simulink model "pathFollowingSystemROS"  (R2020b)
settings: Solver=VariableStepAuto  StartTime=0.0  StopTime=inf  FixedStep=0.01  RelTol=1e-3  EnableMultiTasking=on
PreLoadFcn:
  | load('turtleBotMazeMap.mat')
  | [mapMatrix,mapResolution, mapOrigin] = convertMapToMatrix(myOccMap);
undefined symbols (not defined in the file or in its folder): Angular, Linear, mapMatrix, mapOrigin, mapResolution
libraries: robotlib x4, robotalgslib x2, robotcorelib x1
settings Model: EnablePacing=on  Creator=scastro  LastModifiedBy=josea
settings DataIOCC: LimitDataPoints=on  ReturnWorkspaceOutputs=off
settings OptimizationCC: LifeSpan=inf
settings DebuggingCC: AllowSymbolicDim=off  SFUnexpectedBacktrackingDiag=warning  SFNoUnconditionalDefaultTransitionDiag=warning  SFExecutionAtInitializationDiag=none  ArithmeticOperatorsInVariantConditions=warning
settings SFSimCC: SimUseLocalCustomCode=off  CustomCodeUndefinedFunction=UseInterfaceOnly
settings RTWCC: RTWUseLocalCustomCode=off
settings CodeAppCC: StateflowObjectComments=on
settings GRTTargetCC: TargetLangStandard=C89/C90 (ANSI)
settings ConfigComp: CovMetricSettings=dw  CovSaveCumulativeToWorkspaceVar=on  CovSaveSingleToWorkspaceVar=on  CovExternalEMLEnable=off  CovSFcnEnable=off
settings SimscapeCC: SimscapeNominalValues="[{\"value\":\"10\",\"unit\":\"V\"},{\"value\":\"1\",\"unit\":\"A\"},{\"value\":\"10\",\"unit\":\"N*m\"},{\"value\":\"10\",\"unit\":\"bar\"},{\"value\":\"100\",\"unit\":\"kJ/kg\"},{\"value\":\"1\",\"unit\":\"kW\"},{\"value\":\"300\",\"unit\":\"K\"},{\"value\":\"100\",\"unit\":\"cm^3/s\"},{\"value\":\"1\",\"unit\":\"kN\"},{\"value\":\"1\",\"unit\":\"g/cm^3\"},{\"value\":\"1\",\"unit\":\"l\"},{\"value\":\"1\",\"unit\":\"cm^2\"},{\"value\":\"60\",\"unit\":\"Hz\"}]"  SimscapeLogType=all  SimscapeLogDataHistory=10000
settings ConfigurationSet: Description=SimMechanics 2G
settings ExplorerConfigSet: InternalSimMechanicsExplorerSettings="<ExplorerConfiguration><canonicalview>default</canonicalview><AnimationSetting><BasePlaybackSpeed>1.0</BasePlaybackSpeed><PlaybackSpeedFactor>1.0</PlaybackSpeedFactor></AnimationSetting><TilePanel><TileInfo><Tiles Columns=\"1\" Count=\"1\" Rows=\"1\"><Column Weight=\"1\"/><Row Weight=\"1\"/><Tile Height=\"1\" Width=\"1\" X=\"0\" Y=\"0\"/></Tiles></TileInfo><SceneInfo><SceneViewer><BGColor><R>0.60000002384185791</R><G>0.60000002384185791</G><B>0.60000002384185791</B></BGColor><Camera><DoPerspective>off</DoPerspective><Position><X>-1.70656042355848525</X><Y>-0.974920623359631922</Y><Z>4.72930454537082046</Z></Position><Center><X>0.552860638431633689</X><Y>1.42025063411503494</Y><Z>1.4843509506914252</Z></Center><Up><X>0.664249622453917166</X><Y>0.300615402055903091</Y><Z>0.684399604848363485</Z></Up><ViewLimDist>1</ViewLimDist><YLim>2.77881717169207398</YLim><XLim>3.55928742670435394</XLim></Camera></SceneViewer></SceneInfo></TilePanel><MechEditorPanel><Cameras/><GfxPanelCameraMap/><VideoCreator><PlaybackSpeedRatio>1.0</PlaybackSpeedRatio><FrameRate>30</FrameRate><VideoFormat>Motion JPEG AVI</VideoFormat><FrameSize>auto</FrameSize></VideoCreator></MechEditorPanel></ExplorerConfiguration>"

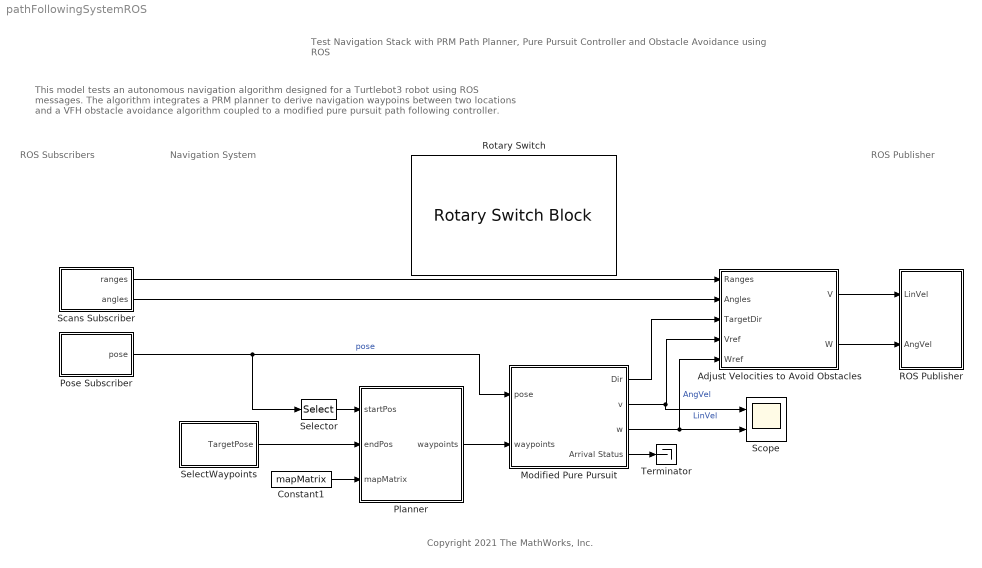
== system pathFollowingSystemROS ==
  note: ROS Publisher
  note: ROS Subscribers
  note: Navigation System
  note: Copyright 2021 The MathWorks, Inc.
  note: Test Navigation Stack with PRM Path Planner, Pure Pursuit Controller and Obstacle Avoidance using ROS
  note: This model tests an autonomous navigation algorithm designed for a Turtlebot3 robot using ROS messages. The algorithm integrates a PRM planner to derive navigation waypoins between two locations and a VFH obstacle avoidance algorithm coupled to a modified pure pursuit path following controller.
  Adjust Velocities to Avoid Obstacles : Subsystem
  Constant1 : Constant  Value=mapMatrix
  Modified Pure Pursuit : Subsystem
  Planner : MATLAB Function  TreatAsAtomicUnit=on  mask{numNodes=50, mapResolution=mapResolution, mapOrigin=mapOrigin, inflateRadius=0.32/2}
      mask prompts: numNodes "Max Number of Nodes"; mapResolution "Map Resolution"; mapOrigin "Map Origin"; inflateRadius "Map Inflate Radius"
  Pose Subscriber : Subsystem
  ROS Publisher : Subsystem
  Rotary Switch : RotarySwitchBlock
      settings: Values={{'Top Right', 'Top Left', 'Bottom Right'}, [1 2 3]}
  Scans Subscriber : Subsystem
  Scope : Scope  NumInputPorts=2
  SelectWaypoints : Subsystem
  Selector : Selector  InputPortWidth=3  IndexOptions=Index vector (dialog)  Indices=[1 2]  OutputSizes=1
  Terminator : Terminator
  wires:
  Modified Pure Pursuit/4(Arrival Status) -> Terminator/1
  Selector/1 -> Planner/1(startPos)
  Constant1/1 -> Planner/3(mapMatrix)
  Planner/1(waypoints) -> Modified Pure Pursuit/2(waypoints)
  Scans Subscriber/1(ranges) -> Adjust Velocities to Avoid Obstacles/1(Ranges)
  Modified Pure Pursuit/1(Dir) -> Adjust Velocities to Avoid Obstacles/3(TargetDir)
  Adjust Velocities to Avoid Obstacles/2(W) -> ROS Publisher/2(AngVel)
  Scans Subscriber/2(angles) -> Adjust Velocities to Avoid Obstacles/2(Angles)
  Modified Pure Pursuit/3(w) -> Scope/2, Adjust Velocities to Avoid Obstacles/5(Wref)  "AngVel"
  Pose Subscriber/1(pose) -> Modified Pure Pursuit/1(pose), Selector/1  "pose"
  Adjust Velocities to Avoid Obstacles/1(V) -> ROS Publisher/1(LinVel)
  Modified Pure Pursuit/2(v) -> Scope/1, Adjust Velocities to Avoid Obstacles/4(Vref)  "LinVel"
  SelectWaypoints/1(TargetPose) -> Planner/2(endPos)

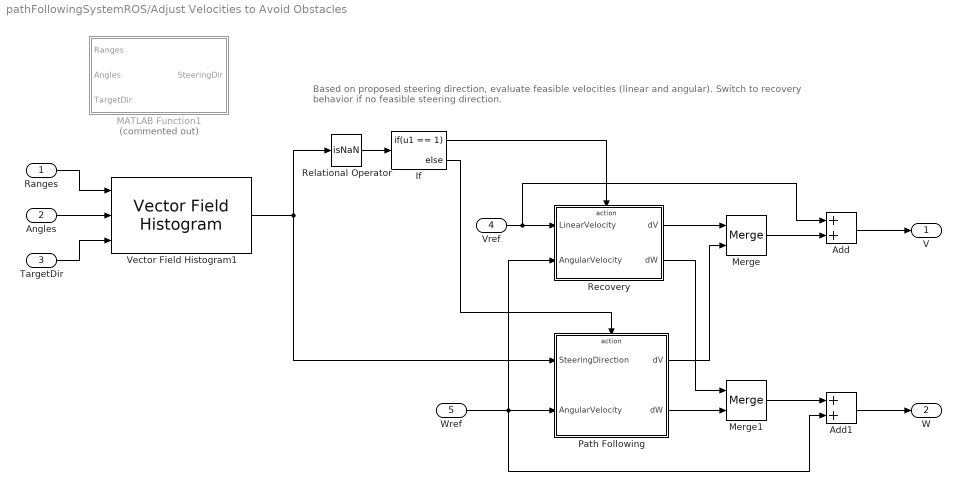
== system pathFollowingSystemROS/Adjust Velocities to Avoid Obstacles ==
  note: Based on proposed steering direction, evaluate feasible velocities (linear and angular).
      | 				Switch to recovery behavior if no feasible steering direction.
  Ranges : Inport
  Angles : Inport  Port=2
  TargetDir : Inport  Port=3
  Vref : Inport  Port=4
  Wref : Inport  Port=5
  Add : Sum
  Add1 : Sum
  If : If  IfExpression=u1 == 1
  MATLAB Function1 : MATLAB Function  Commented=on  TreatAsAtomicUnit=on
  Merge : Merge
  Merge1 : Merge
  Path Following : Subsystem  TreatAsAtomicUnit=on
  Recovery : Subsystem  TreatAsAtomicUnit=on
  Relational Operator : RelationalOperator  Operator=isNaN  OutDataTypeStr=boolean  RndMeth=Simplest
  Vector Field Histogram1 : robotalgslib/Vector Field Histogram  NumAngularSectors=180  DistanceLimits=[ 0.05, 2 ]  HistogramThresholds=[ 0.5, 7 ]  RobotRadius=0.15  SafetyDistance=0.08  MinTurningRadius=0.1  SimulateUsing=Code generation  TargetDirectionWeight=7  CurrentDirectionWeight=2  PreviousDirectionWeight=2
      settings: SourceProductBaseCode=NV,RO
  V : Outport  VectorParamsAs1DForOutWhenUnconnected=off
  W : Outport  Port=2  VectorParamsAs1DForOutWhenUnconnected=off
  wires:
  Vref/1 -> Add/1, Recovery/1(LinearVelocity)
  Vector Field Histogram1/1 -> Relational Operator/1, Path Following/1(SteeringDirection)
  Wref/1 -> Add1/2, Recovery/2(AngularVelocity), Path Following/2(AngularVelocity)
  Relational Operator/1 -> If/1
  Angles/1 -> Vector Field Histogram1/2
  TargetDir/1 -> Vector Field Histogram1/3
  If/1 -> Recovery/Action
  If/2 -> Path Following/Action
  Recovery/2(dW) -> Merge1/1
  Path Following/2(dW) -> Merge1/2
  Recovery/1(dV) -> Merge/1
  Path Following/1(dV) -> Merge/2
  Merge1/1 -> Add1/1
  Merge/1 -> Add/2
  Ranges/1 -> Vector Field Histogram1/1
  Add1/1 -> W/1
  Add/1 -> V/1

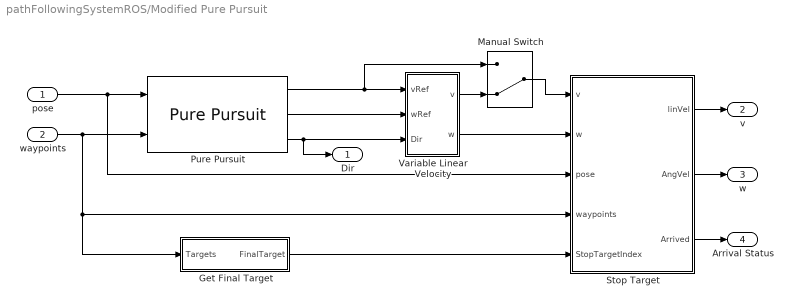
== system pathFollowingSystemROS/Modified Pure Pursuit ==
  pose : Inport
  waypoints : Inport  Port=2
  Get Final Target : Subsystem
  Manual Switch : ManualSwitch  CurrentSetting=0
  Pure Pursuit : robotalgslib/Pure Pursuit  DesiredLinearVelocity=0.15 %0.26  MaxAngularVelocity=1.82  LookaheadDistance=0.5  TargetDirPort=on  SimulateUsing=Code generation
  Stop Target : Subsystem  mask(Stop at Target){threshold=0.8}
      mask prompts: threshold "Threshold Radius"
      mask help: This block takes in robot commands and a set of waypoints to set a velocity of zero when the robot pose compared to the waypoint is within the threshold specified.
  Variable Linear Velocity : Subsystem  mask(Steer-Proportional Linear Velocity){pGain=1, deadZone=pi/8}
      mask prompts: pGain "Turn Slow-Down Factor"; deadZone "Target Direction Deadzone"
      mask help: This block reduces the linear velocity of the robot with respect to the target direction in order to reach the desired waypoints more accurately.
  Dir : Outport  VectorParamsAs1DForOutWhenUnconnected=off
  v : Outport  Port=2  VectorParamsAs1DForOutWhenUnconnected=off
  w : Outport  Port=3  VectorParamsAs1DForOutWhenUnconnected=off
  Arrival Status : Outport  Port=4  VectorParamsAs1DForOutWhenUnconnected=off
  wires:
  pose/1 -> Pure Pursuit/1, Stop Target/3(pose)
  waypoints/1 -> Stop Target/4(waypoints), Get Final Target/1(Targets), Pure Pursuit/2
  Stop Target/3(Arrived) -> Arrival Status/1
  Stop Target/1(linVel) -> v/1
  Stop Target/2(AngVel) -> w/1
  Get Final Target/1(FinalTarget) -> Stop Target/5(StopTargetIndex)
  Pure Pursuit/1 -> Manual Switch/1, Variable Linear Velocity/1(vRef)
  Variable Linear Velocity/2(w) -> Stop Target/2(w)
  Pure Pursuit/2 -> Variable Linear Velocity/2(wRef)
  Pure Pursuit/3 -> Dir/1, Variable Linear Velocity/3(Dir)
  Variable Linear Velocity/1(v) -> Manual Switch/2
  Manual Switch/1 -> Stop Target/1(v)

== system pathFollowingSystemROS/Pose Subscriber ==
  Extract Pose : Subsystem
  Subscribe : robotlib/Subscribe  topicSource=Select from ROS network  topic=/odom  messageType=nav_msgs/Odometry  SampleTime=0.02  legacyBusStruct=off  messageQueueLength=1
  pose : Outport
  wires:
  Subscribe/2 -> Extract Pose/1(odom)
  Subscribe/1 -> Extract Pose/Enable
  Extract Pose/1(pose) -> pose/1

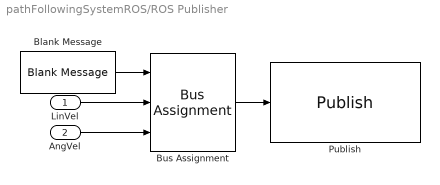
== system pathFollowingSystemROS/ROS Publisher ==
  LinVel : Inport
  AngVel : Inport  Port=2
  Blank Message : robotlib/Blank Message  messageClass=Message  entityType=geometry_msgs/Twist  messageType=geometry_msgs/Twist  SampleTime=inf  legacyBusStruct=off
  Bus Assignment : BusAssignment  AssignedSignals=Linear.X,Angular.Z
  Publish : robotlib/Publish  topicSource=Select from ROS network  topic=/cmd_vel  messageType=geometry_msgs/Twist  legacyBusStruct=off  messageQueueLength=1
  wires:
  Bus Assignment/1 -> Publish/1
  Blank Message/1 -> Bus Assignment/1
  LinVel/1 -> Bus Assignment/2
  AngVel/1 -> Bus Assignment/3

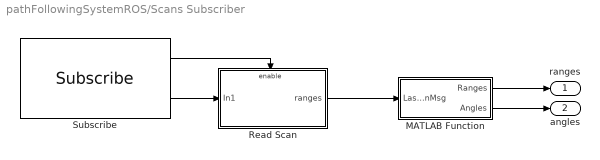
== system pathFollowingSystemROS/Scans Subscriber ==
  MATLAB Function : MATLAB Function  TreatAsAtomicUnit=on
  Read Scan : Subsystem
  Subscribe : robotlib/Subscribe  topicSource=Select from ROS network  topic=/scan  messageType=sensor_msgs/LaserScan  SampleTime=0.02  legacyBusStruct=off  messageQueueLength=1
  ranges : Outport
  angles : Outport  Port=2
  wires:
  Subscribe/1 -> Read Scan/Enable
  Subscribe/2 -> Read Scan/1(In1)
  Read Scan/1(ranges) -> MATLAB Function/1(LaserScanMsg)
  MATLAB Function/1(Ranges) -> ranges/1
  MATLAB Function/2(Angles) -> angles/1

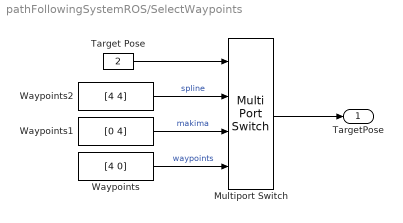
== system pathFollowingSystemROS/SelectWaypoints ==
  Multiport Switch : MultiPortSwitch
  Target Pose : Constant  Value=2
  Waypoints : Constant  Value=[4 0]
  Waypoints1 : Constant  Value=[0 4]
  Waypoints2 : Constant  Value=[4 4]
  TargetPose : Outport
  wires:
  Multiport Switch/1 -> TargetPose/1
  Waypoints/1 -> Multiport Switch/4  "waypoints"
  Waypoints1/1 -> Multiport Switch/3  "makima"
  Waypoints2/1 -> Multiport Switch/2  "spline"
  Target Pose/1 -> Multiport Switch/1

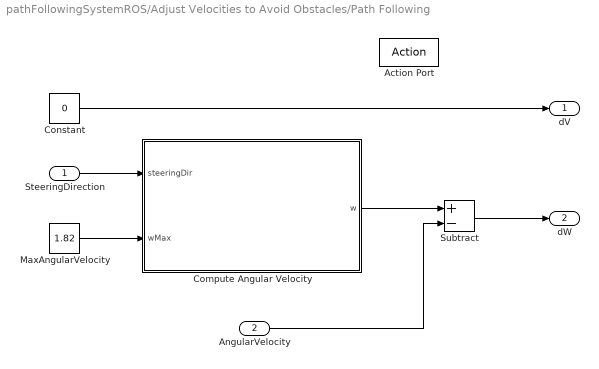
== system pathFollowingSystemROS/Adjust Velocities to Avoid Obstacles/Path Following ==
  SteeringDirection : Inport
  AngularVelocity : Inport  Port=2
  Action Port : ActionPort  ActionPortLabel=else
  Compute Angular Velocity : MATLAB Function  TreatAsAtomicUnit=on
  Constant : Constant  Value=0
  MaxAngularVelocity : Constant  Value=1.82
  Subtract : Sum  Inputs=+-
  dV : Outport  VectorParamsAs1DForOutWhenUnconnected=off
  dW : Outport  Port=2  VectorParamsAs1DForOutWhenUnconnected=off
  wires:
  Constant/1 -> dV/1
  MaxAngularVelocity/1 -> Compute Angular Velocity/2(wMax)
  SteeringDirection/1 -> Compute Angular Velocity/1(steeringDir)
  Subtract/1 -> dW/1
  Compute Angular Velocity/1(w) -> Subtract/1
  AngularVelocity/1 -> Subtract/2

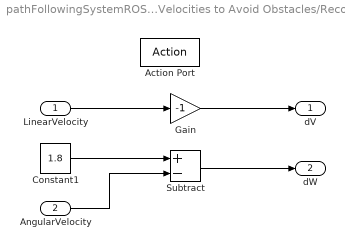
== system pathFollowingSystemROS/Adjust Velocities to Avoid Obstacles/Recovery ==
  LinearVelocity : Inport
  AngularVelocity : Inport  Port=2
  Action Port : ActionPort  ActionPortLabel=if(u1 == 1)
  Constant1 : Constant  Value=1.8
  Gain : Gain  Gain=-1
  Subtract : Sum  Inputs=+-
  dV : Outport  VectorParamsAs1DForOutWhenUnconnected=off
  dW : Outport  Port=2  VectorParamsAs1DForOutWhenUnconnected=off
  wires:
  LinearVelocity/1 -> Gain/1
  Gain/1 -> dV/1
  Constant1/1 -> Subtract/1
  AngularVelocity/1 -> Subtract/2
  Subtract/1 -> dW/1

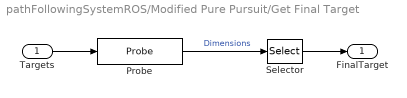
== system pathFollowingSystemROS/Modified Pure Pursuit/Get Final Target ==
  Targets : Inport
  Probe : Probe  ProbeWidth=off  ProbeSampleTime=off  ProbeComplexSignal=off  ProbeSignalDimensions=on
  Selector : Selector  InputPortWidth=2  IndexOptions=Index vector (dialog)  Indices=1  OutputSizes=1
  FinalTarget : Outport
  wires:
  Probe/1 -> Selector/1  "Dimensions"
  Selector/1 -> FinalTarget/1
  Targets/1 -> Probe/1

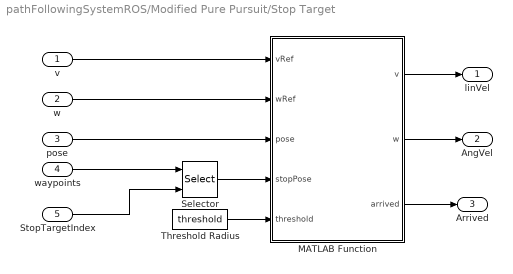
== system pathFollowingSystemROS/Modified Pure Pursuit/Stop Target ==
  v : Inport
  w : Inport  Port=2
  pose : Inport  Port=3
  waypoints : Inport  Port=4
  StopTargetIndex : Inport  Port=5
  MATLAB Function : MATLAB Function  TreatAsAtomicUnit=on
  Selector : Selector  NumberOfDimensions=2  InputPortWidth=3  IndexOptions=Index vector (port),Index vector (dialog)  Indices=[1 3],[1 2]  OutputSizes=1,1
  Threshold Radius : Constant  Value=threshold
  linVel : Outport
  AngVel : Outport  Port=2
  Arrived : Outport  Port=3
  wires:
  v/1 -> MATLAB Function/1(vRef)
  Selector/1 -> MATLAB Function/4(stopPose)
  StopTargetIndex/1 -> Selector/2
  waypoints/1 -> Selector/1
  MATLAB Function/1(v) -> linVel/1
  pose/1 -> MATLAB Function/3(pose)
  w/1 -> MATLAB Function/2(wRef)
  Threshold Radius/1 -> MATLAB Function/5(threshold)
  MATLAB Function/3(arrived) -> Arrived/1
  MATLAB Function/2(w) -> AngVel/1

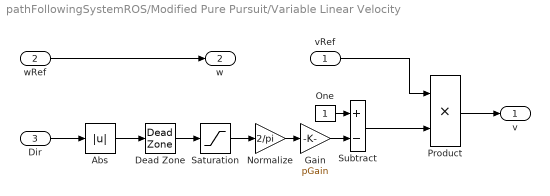
== system pathFollowingSystemROS/Modified Pure Pursuit/Variable Linear Velocity ==
  vRef : Inport
  wRef : Inport  Port=2
  Dir : Inport  Port=3
  Abs : Abs
  Dead Zone : DeadZone  LowerValue=-deadZone  UpperValue=deadZone  SaturateOnIntegerOverflow=on
  Gain : Gain  Gain=pGain
  Normalize : Gain  Gain=2/pi
  One : Constant  OutDataTypeStr=Inherit: Inherit via back propagation
  Product : Product
  Saturation : Saturate  UpperLimit=pi/2  LowerLimit=0
  Subtract : Sum  Inputs=+-
  v : Outport
  w : Outport  Port=2
  wires:
  Dir/1 -> Abs/1
  One/1 -> Subtract/1
  wRef/1 -> w/1
  vRef/1 -> Product/1
  Abs/1 -> Dead Zone/1
  Saturation/1 -> Normalize/1
  Subtract/1 -> Product/2
  Normalize/1 -> Gain/1
  Gain/1 -> Subtract/2
  Dead Zone/1 -> Saturation/1
  Product/1 -> v/1

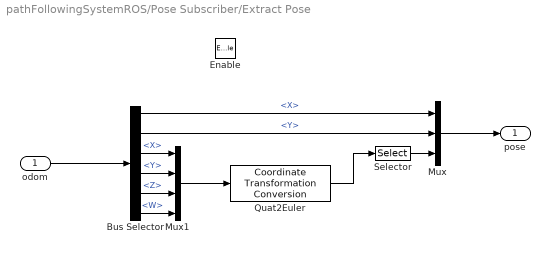
== system pathFollowingSystemROS/Pose Subscriber/Extract Pose ==
  odom : Inport
  Enable : EnablePort
  Bus Selector : BusSelector  OutputSignals=Pose.Pose.Position.X,Pose.Pose.Position.Y,Pose.Pose.Orientation.X,Pose.Pose.Orientation.Y,Pose.Pose.Orientation.Z,Pose.Pose.Orientation.W
  Mux : Mux  Inputs=3
  Mux1 : Mux
  Quat2Euler : robotcorelib/Coordinate Transformation Conversion  InputRepresentation=Quaternion  InputEulerSequence=ZYX  ShowTrVecInputPort=on  OutputRepresentation=Euler Angles  OutputEulerSequence=ZYX  ShowTrVecOutputPort=on  SimulateUsing=Interpreted execution
      settings: SourceProductBaseCode=NV,RO,RR,UV
  Selector : Selector  InputPortWidth=3  IndexOptions=Index vector (dialog)  Indices=3  OutputSizes=1
  pose : Outport
  wires:
  Quat2Euler/1 -> Selector/1
  Bus Selector/5 -> Mux1/3  "<Z>"
  Selector/1 -> Mux/3
  Mux1/1 -> Quat2Euler/1
  Bus Selector/2 -> Mux/2  "<Y>"
  Bus Selector/6 -> Mux1/4  "<W>"
  Bus Selector/1 -> Mux/1  "<X>"
  Bus Selector/3 -> Mux1/1  "<X>"
  Bus Selector/4 -> Mux1/2  "<Y>"
  odom/1 -> Bus Selector/1
  Mux/1 -> pose/1

== system pathFollowingSystemROS/Scans Subscriber/Read Scan ==
  In1 : Inport
  Enable : EnablePort
  ranges : Outport
  wires:
  In1/1 -> ranges/1

== matlab function pathFollowingSystemROS/Planner ==
  settings: updateMethod=DISCRETE
  data: startPos input size=[1 2]; endPos input size=[1 2]; waypoints output size=[50 2]; mapMatrix input; mapResolution parameter; mapOrigin parameter; inflateRadius parameter
function waypoints = PRM_codegen(startPos, endPos, mapMatrix, mapResolution, mapOrigin, inflateRadius)

persistent waypointsInternal
persistent prevStartPos
persistent prevEndPos

% Set constant parameters
maxNumNodes = 50;

% Initialize persistent variables that are used downstream
if isempty(prevStartPos)
    prevStartPos = startPos;
end

if isempty(prevEndPos)
    prevEndPos = endPos;
end

isNewPath = (~isequal(prevEndPos, endPos));

if isempty(waypointsInternal) || isNewPath
    % Two conditions in which waypoints must be set: they are not yet
    % initialized, or they are initialized, but the current start and end
    % do not match those used to generate the previous set of waypoints
    [waypointsInternal] = planPath(mapMatrix, maxNumNodes, startPos, endPos, mapResolution);
end

% Update the outputs
waypoints = waypointsInternal;

% Update the persistent variables that indicate previous state
prevStartPos = startPos;
prevEndPos = endPos;

%% Helper Function

function wayPoints = planPath(mapMatrix, maxNodes, startPos, endPos, mapResolution)
    % Offset points according to Map Origin
    startPos = startPos - mapOrigin;
    endPos = endPos - mapOrigin;
    % Create a probabilistic roadmap
    map = binaryOccupancyMap(mapMatrix, mapResolution);
    inflate(map,inflateRadius);
    prm = mobileRobotPRM(map, maxNodes);
    % show(prm)
    % Find a path between two points
    xy = findpath(prm, startPos(:)', endPos(:)');
 
    %wayPoints = repmat(endPos(:)', maxNodes, 1);
    wayPoints = xy +repmat(mapOrigin,length(xy),1);
    % Number of nodes that are actually used
    %numNodes = length(xy);
    %wayPoints(1:numNodes,:) = xy;    

end

end

== matlab function pathFollowingSystemROS/Adjust Velocities to Avoid Obstacles/Path Following/Compute Angular Velocity ==
  data: steeringDir input; w output; wMax input
function w = exampleHelperComputeAngularVelocity(steeringDir, wMax)
%EXAMPLEHELPERCOMPUTEANGULARVELOCITY Compute angular velocity
%   W = exampleHelperComputeAngularVelocity(STEERINGDIR)
%   returns the angular velocity W for a differential drive robot in radians
%   per second for a given steering direction STEERINGDIR in the robot's
%   coordinate frame in radians.
%
%   W = exampleHelperComputeAngularVelocity(STEERINGDIR, WMAX)
%   returns the angular velocity W for a differential drive robot in radians
%   per second for a given steering direction STEERINGDIR in the robot's
%   coordinate frame in radians and maximum angular velocity WMAX in
%   radians per second. The output angular velocity is saturated based on
%   the WMAX.
%
%   Example:
%       
%       w = exampleHelperComputeAngularVelocity(0.2, 1);

% Copyright 2015 The MathWorks, Inc.

%#codegen
%#ok<*EMCA>

% Allow variable input arguments
if nargin == 1   
    wMax = inf;
end

validateattributes(steeringDir, {'double'},{'real'},...
    'exampleHelperComputeAngularVelocity', 'STEERINGDIR', 1);
validateattributes(wMax, {'double'},{'real', 'positive'},...
    'exampleHelperComputeAngularVelocity', 'WMAX', 2);

% Computing in robot's coordinate frame
curPose = [0 0 0];

% The following computation is similar to robotics.PurePursuit
lookaheadPoint = [cos(steeringDir), sin(steeringDir)];
slope = atan2((lookaheadPoint(2) - curPose(2)), ...
    (lookaheadPoint(1) - curPose(1)));
alpha = angdiff(curPose(3), slope);

% Angular velocity command for a differential drive robot is
% equal to the desired curvature to be followed by the robot.

w = (2*sin(alpha));

% Pick a constant rotation when robot is facing in the opposite
% direction of the path
if abs(abs(alpha) - pi) < 1e-12
    w = sign(w)*1;
end

if abs(w) > wMax
    w = sign(w)*wMax;
end

end

== matlab function pathFollowingSystemROS/Modified Pure Pursuit/Stop Target/MATLAB Function ==
  data: v output; w output; vRef input; wRef input; pose input; stopPose input; threshold input; arrived output
function [v, w, arrived] = arrivalThreshold(vRef, wRef, pose, stopPose, threshold)

eucDist = sqrt((stopPose(1)-pose(1))^2 + (stopPose(2)-pose(2))^2);

if eucDist > threshold
    v = vRef;
    w = wRef;
    arrived = 0;
else
    v = 0;
    w = 0;
    arrived = 1;
end

== matlab function pathFollowingSystemROS/Adjust Velocities to Avoid Obstacles/MATLAB Function1 ==
  data: SteeringDir output; Ranges input; Angles input; TargetDir input
function SteeringDir = fcn(Ranges, Angles, TargetDir)
SteeringDir = 0;
coder.extrinsic('vizVFH')
SteeringDir = vizVFH(Ranges,Angles,TargetDir);

== matlab function pathFollowingSystemROS/Scans Subscriber/MATLAB Function ==
  data: LaserScanMsg input; Ranges output; Angles output
function [Ranges, Angles] = ExtractRangeData(LaserScanMsg)
%#codegen

% Extract Range information
Ranges = double(LaserScanMsg.Ranges);

% Construct Angles vector using AngleMin and AngleIncrement from sensor
% reading.
angMin = double(LaserScanMsg.AngleMin);
angIncrement = double(LaserScanMsg.AngleIncrement);

numReadings = numel(Ranges);
rawAngles = angMin + (0:numReadings-1)' * angIncrement;

% Wrap the angles to the (-pi,pi] interval.
Angles = robotics.internal.wrapToPi(double(rawAngles));
